simulink model "PubIfControlLONC_MDL"  (R2020b)
settings: configuration reference "DspaceConfig" (kept outside this file)
PostLoadFcn:
  | if any(exist('dsrtsu_mdlpostloadfcn', 'file') ~= 0), dsrtsu_mdlpostloadfcn('Execute', bdroot); end
InitFcn:
  | , if any(exist('rtifpga_mdlclblib', 'file') ~= 0), rtifpga_mdlclblib('Init', bdroot); end,
  | , if any(exist('dsmpb_private', 'file') ~= 0), dsmpb_private('dsmpb_mdlclblib', 'Init', bdroot); end,
PreSaveFcn:
  | , if any(exist('dsmpb_private', 'file') ~= 0), dsmpb_private('dsmpb_mdlclblib', 'PreSave', bdroot); end,
CloseFcn:
  | , if any(exist('dsmpb_private', 'file') ~= 0), dsmpb_private('dsmpb_mdlclblib', 'Close', bdroot); end,
settings Model: DataDictionary=HWA_DDs.sldd  RTICANMMDATA=struct('GeneralSetupData',struct('modelroot','D:\10_HWA_Project\Git_ADAS_Store\Adas\LONC','generalsettings',struct('filesettings',struct('destfolder',struct('Name','RTICANMM_FILES','Check',1),'buildfolder',struct('Name','.','Check',1),'AbsDestfolder',struct('Name','D:\10_HWA_Project\Git_ADAS_Store\Adas\LONC\RTICANMM_FILES'),'AbsBuildfolder',struct('Name','D:\10_HWA_Project\Git_ADAS_Store\Adas\LONC'))),'options',struct('addpaths',1,'rmpaths',1,'addtrcexclusion',false,'cannavigator',struct('checkmonitoring',0),'show_usrtrc',0,'use_usrtrc',0),'advanced',struct('options',ones(1,100)),'MPSetup',{{}},'RTI',struct('Type','DSRT','Ver','4.4','Date','02-Nov-2020'),'modelname','PubIfControlLONC_MDL','block','PubIfControlLONC_MDL'))  DSRTSU_INTERNAL_RTIFPGA=170  Creator=GW00180895  LastModifiedBy=GW00201118
settings ConfigSetRef: SourceName=DspaceConfig

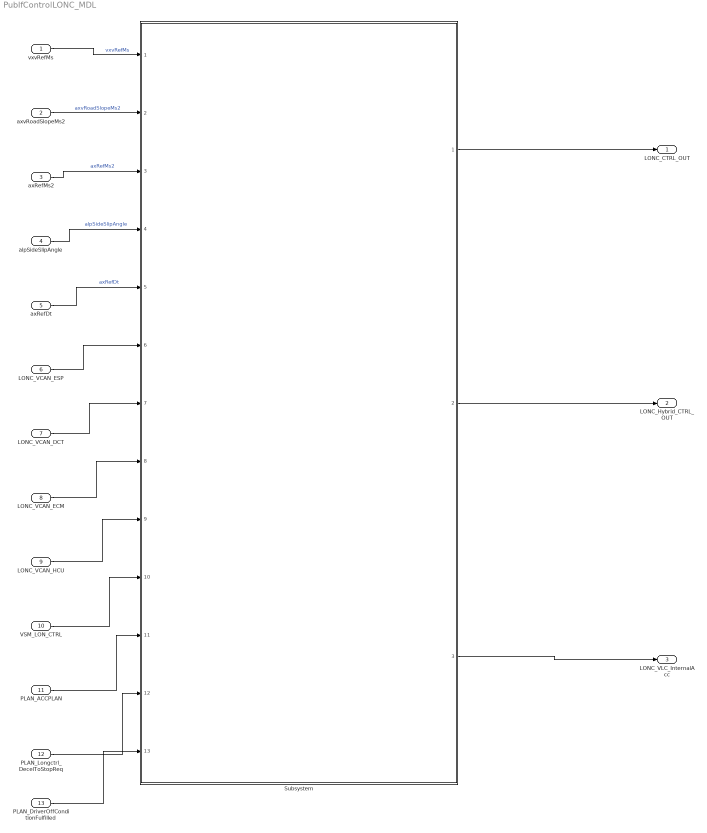
== system PubIfControlLONC_MDL ==
  vxvRefMs : Inport  OutDataTypeStr=single  PortDimensions=1  BusOutputAsStruct=on
  axvRoadSlopeMs2 : Inport  Port=2  OutDataTypeStr=single  PortDimensions=1  BusOutputAsStruct=on
  axRefMs2 : Inport  Port=3  OutDataTypeStr=single  PortDimensions=1  BusOutputAsStruct=on
  alpSideSlipAngle : Inport  Port=4  OutDataTypeStr=single  PortDimensions=1  BusOutputAsStruct=on
  axRefDt : Inport  Port=5  OutDataTypeStr=single  PortDimensions=1  BusOutputAsStruct=on
  LONC_VCAN_ESP : Inport  Port=6  OutDataTypeStr=Bus: VCAN_ESP_MSG_BUS  PortDimensions=1  BusOutputAsStruct=on
  LONC_VCAN_DCT : Inport  Port=7  OutDataTypeStr=Bus: VCAN_DCT_MSG_BUS  PortDimensions=1  BusOutputAsStruct=on
  LONC_VCAN_ECM : Inport  Port=8  OutDataTypeStr=Bus: VCAN_ECM_MSG_BUS  PortDimensions=1  BusOutputAsStruct=on
  LONC_VCAN_HCU : Inport  Port=9  OutDataTypeStr=Bus: VCAN_HCU_MSG_BUS  PortDimensions=1  BusOutputAsStruct=on
  VSM_LON_CTRL : Inport  Port=10  OutDataTypeStr=Bus: VSM_LON_CTRL_BUS  PortDimensions=1  BusOutputAsStruct=on
  PLAN_ACCPLAN : Inport  Port=11  OutDataTypeStr=Bus: PLAN_ACCPLAN_BUS
  PLAN_Longctrl_DecelToStopReq : Inport  Port=12  OutDataTypeStr=boolean  PortDimensions=1  BusOutputAsStruct=on
  PLAN_DriverOffConditionFulfilled : Inport  Port=13  OutDataTypeStr=boolean  PortDimensions=1  BusOutputAsStruct=on
  Subsystem : Subsystem  ReferencedSubsystem=PvtSubSys_LONC
  LONC_CTRL_OUT : Outport  OutDataTypeStr=Bus: LONC_CTRL_OUT_BUS  PortDimensions=1  BusOutputAsStruct=on
  LONC_Hybrid_CTRL_OUT : Outport  Port=2  OutDataTypeStr=Bus: LONC_Hybrid_CTRL_OUT_BUS  PortDimensions=1  BusOutputAsStruct=on
  LONC_VLC_InternalAcc : Outport  Port=3  OutDataTypeStr=single
  wires:
  vxvRefMs/1 -> Subsystem/1  "vxvRefMs"
  axvRoadSlopeMs2/1 -> Subsystem/2  "axvRoadSlopeMs2"
  axRefMs2/1 -> Subsystem/3  "axRefMs2"
  alpSideSlipAngle/1 -> Subsystem/4  "alpSideSlipAngle"
  axRefDt/1 -> Subsystem/5  "axRefDt"
  LONC_VCAN_ESP/1 -> Subsystem/6
  LONC_VCAN_DCT/1 -> Subsystem/7
  LONC_VCAN_ECM/1 -> Subsystem/8
  LONC_VCAN_HCU/1 -> Subsystem/9
  VSM_LON_CTRL/1 -> Subsystem/10
  PLAN_ACCPLAN/1 -> Subsystem/11
  PLAN_Longctrl_DecelToStopReq/1 -> Subsystem/12
  Subsystem/1 -> LONC_CTRL_OUT/1
  Subsystem/2 -> LONC_Hybrid_CTRL_OUT/1
  Subsystem/3 -> LONC_VLC_InternalAcc/1
  PLAN_DriverOffConditionFulfilled/1 -> Subsystem/13
